simulink model "lineaEEC_prom"  (R2015a)
settings: Solver=ode45  StartTime=0.0  StopTime=0.1  RelTol=1e-3
values from neighbouring files (symbols this model uses):
  l0 = (0.002029 + 0.002392 + 0.002727 + 0.002296)/4    (= 0.002361)    [ParametrosTramo1.m]
  l1 = (0.001327 + 0.001263 + 0.001096 + 0.001311)/4    (= 0.00124925)    [ParametrosTramo1.m]
  Long = [0.26386 9.910026 3.09144 7.97976 2.97622 3.41433 1.495 4.41558 3.73037 10.41391 7.695292 4.39497 8.025209 3.99747 5.70753 10.31599 7.45101]'    [ParametrosTramo1.m]
  r0 = (0.4148+0.8307*3)/4    (= 0.726725)    [ParametrosTramo1.m]
  r1 = (0.4153+0.8315*3)/4    (= 0.72745)    [ParametrosTramo1.m]
libraries: powerlib x96
settings Model: CovSFcnEnable=off  Creator=ricardo  LastModifiedBy=USUARIO
settings DebuggingCC: SolverPrmCheckMsg=warning

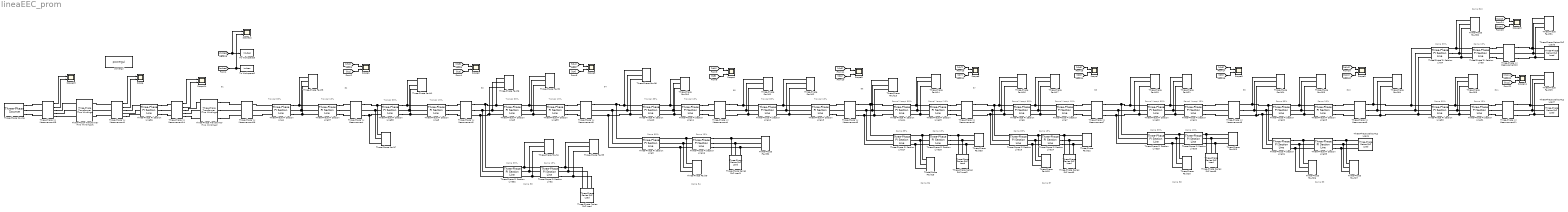
== system lineaEEC_prom ==
  note: B11
  note: B10
  note: B9
  note: B8
  note: B7
  note: B6
  note: B5
  note: B4
  note: Rama B3
  note: B3
  note: B2
  note: B1
  note: Rama 85%
  note: Troncal 85%
  note: Troncal 15%
  note: Rama 15%
  note: Troncal 85%
  note: Troncal 15%
  note: Troncal 85%
  note: Troncal 15%
  note: Troncal 85%
  note: Troncal 15%
  note: Troncal 85%
  note: Troncal 15%
  note: Rama 85%
  note: Rama 15%
  note: Rama 85%
  note: Rama 15%
  note: Ramal Yacopi 85%
  note: Ramal Yacopi 15%
  note: Ramal Yacopi 85%
  note: Ramal Yacopi 15%
  note: Ramal Yacopi 85%
  note: Ramal Yacopi 15%
  note: Rama 85%
  note: Rama 15%
  note: Rama 85%
  note: Rama 15%
  note: Rama 85%
  note: Rama 15%
  note: Rama 85%
  note: Rama 15%
  note: Rama 85%
  note: Rama 15%
  note: Rama B4
  note: Rama B6
  note: Rama B7
  note: Rama B8
  note: Rama B9
  note: Rama B10
  Scope{,1..12,14..15} (15 alike) : Scope  NumInputPorts=2
      Scope settings: YMin=-5~-5  YMax=5~5
      Scope1 settings: YMin=-5~-5  YMax=5~5
      Scope10 settings: YMin=-5~-5  YMax=5~5  SaveName=ScopeData10
      Scope11 settings: YMin=-5~-5  YMax=5~5  SaveName=ScopeData11
      Scope12 settings: TimeRange=0.03177083333333333  YMin=-4000~-5  YMax=4000~5  SaveName=ScopeData12
      Scope14 settings: YMin=-5~-5  YMax=5~5  SaveName=ScopeData14
      Scope15 settings: YMin=-175000~-1  YMax=100000~1.1  SaveName=ScopeData15
      Scope2 settings: YMin=-5~-5  YMax=5~5  SaveName=ScopeData2
      Scope3 settings: YMin=-5~-5  YMax=5~5  SaveName=ScopeData3
      Scope4 settings: YMin=-5~-5  YMax=5~5  SaveName=ScopeData4
      Scope5 settings: YMin=-5~-5  YMax=5~5  SaveName=ScopeData5
      Scope6 settings: YMin=-5~-5  YMax=5~5  SaveName=ScopeData6
      Scope7 settings: YMin=-5~-5  YMax=5~5  SaveName=ScopeData7
      Scope8 settings: YMin=-5~-5  YMax=5~5  SaveName=ScopeData8
      Scope9 settings: YMin=-5~-5  YMax=5~5  SaveName=ScopeData9
  Three-Phase PI Section Line1 : powerlib/Elements/Three-Phase PI Section Line  LConnTagsString=a|b|c  RConnTagsString=A|B|C  Frequency=60  Resistances=[ r1 r0]  Inductances="[ l1  l0]"  Capacitances=[12.74e-9 7.751e-9]  Length=Long(1)/2
  Three-Phase PI Section Line10 : powerlib/Elements/Three-Phase PI Section Line  LConnTagsString=a|b|c  RConnTagsString=A|B|C  Frequency=60  Resistances=[ r1 r0]  Inductances="[ l1  l0]"  Capacitances=[12.74e-9 7.751e-9]  Length=Long(4)/2
  Three-Phase PI Section Line11 : powerlib/Elements/Three-Phase PI Section Line  LConnTagsString=a|b|c  RConnTagsString=A|B|C  Frequency=60  Resistances=[ r1 r0]  Inductances="[ l1  l0]"  Capacitances=[12.74e-9 7.751e-9]  Length=Long(4)/2
  Three-Phase PI Section Line12 : powerlib/Elements/Three-Phase PI Section Line  LConnTagsString=a|b|c  RConnTagsString=A|B|C  Frequency=60  Resistances=[ r1 r0]  Inductances="[ l1  l0]"  Capacitances=[12.74e-9 7.751e-9]  Length=Long(5)/2
  Three-Phase PI Section Line13 : powerlib/Elements/Three-Phase PI Section Line  LConnTagsString=a|b|c  RConnTagsString=A|B|C  Frequency=60  Resistances=[ r1 r0]  Inductances="[ l1  l0]"  Capacitances=[12.74e-9 7.751e-9]  Length=Long(5)/2
  Three-Phase PI Section Line14 : powerlib/Elements/Three-Phase PI Section Line  LConnTagsString=a|b|c  RConnTagsString=A|B|C  Frequency=60  Resistances=[ r1 r0]  Inductances="[ l1  l0]"  Capacitances=[12.74e-9 7.751e-9]  Length=Long(6)/2
  Three-Phase PI Section Line15 : powerlib/Elements/Three-Phase PI Section Line  LConnTagsString=a|b|c  RConnTagsString=A|B|C  Frequency=60  Resistances=[ r1 r0]  Inductances="[ l1  l0]"  Capacitances=[12.74e-9 7.751e-9]  Length=Long(6)/2
  Three-Phase PI Section Line16 : powerlib/Elements/Three-Phase PI Section Line  LConnTagsString=a|b|c  RConnTagsString=A|B|C  Frequency=60  Resistances=[ r1 r0]  Inductances="[ l1  l0]"  Capacitances=[12.74e-9 7.751e-9]  Length=Long(12)/2
  Three-Phase PI Section Line17 : powerlib/Elements/Three-Phase PI Section Line  LConnTagsString=a|b|c  RConnTagsString=A|B|C  Frequency=60  Resistances=[ r1 r0]  Inductances="[ l1  l0]"  Capacitances=[12.74e-9 7.751e-9]  Length=Long(13)/2
  Three-Phase PI Section Line18 : powerlib/Elements/Three-Phase PI Section Line  LConnTagsString=a|b|c  RConnTagsString=A|B|C  Frequency=60  Resistances=[ r1 r0]  Inductances="[ l1  l0]"  Capacitances=[12.74e-9 7.751e-9]  Length=Long(13)/2
  Three-Phase PI Section Line19 : powerlib/Elements/Three-Phase PI Section Line  LConnTagsString=a|b|c  RConnTagsString=A|B|C  Frequency=60  Resistances=[ r1 r0]  Inductances="[ l1  l0]"  Capacitances=[12.74e-9 7.751e-9]  Length=Long(14)/2
  Three-Phase PI Section Line2 : powerlib/Elements/Three-Phase PI Section Line  LConnTagsString=a|b|c  RConnTagsString=A|B|C  Frequency=60  Resistances=[ r1 r0]  Inductances="[ l1  l0]"  Capacitances=[12.74e-9 7.751e-9]  Length=Long(11)/2
  Three-Phase PI Section Line20 : powerlib/Elements/Three-Phase PI Section Line  LConnTagsString=a|b|c  RConnTagsString=A|B|C  Frequency=60  Resistances=[ r1 r0]  Inductances="[ l1  l0]"  Capacitances=[12.74e-9 7.751e-9]  Length=Long(8)/2
  Three-Phase PI Section Line21 : powerlib/Elements/Three-Phase PI Section Line  LConnTagsString=a|b|c  RConnTagsString=A|B|C  Frequency=60  Resistances=[ r1 r0]  Inductances="[ l1  l0]"  Capacitances=[12.74e-9 7.751e-9]  Length=Long(8)/2
  Three-Phase PI Section Line22 : powerlib/Elements/Three-Phase PI Section Line  LConnTagsString=a|b|c  RConnTagsString=A|B|C  Frequency=60  Resistances=[ r1 r0]  Inductances="[ l1  l0]"  Capacitances=[12.74e-9 7.751e-9]  Length=Long(9)/2
  Three-Phase PI Section Line23 : powerlib/Elements/Three-Phase PI Section Line  LConnTagsString=a|b|c  RConnTagsString=A|B|C  Frequency=60  Resistances=[ r1 r0]  Inductances="[ l1  l0]"  Capacitances=[12.74e-9 7.751e-9]  Length=Long(9)/2
  Three-Phase PI Section Line24 : powerlib/Elements/Three-Phase PI Section Line  LConnTagsString=a|b|c  RConnTagsString=A|B|C  Frequency=60  Resistances=[ r1 r0]  Inductances="[ l1  l0]"  Capacitances=[12.74e-9 7.751e-9]  Length=Long(14)/2
  Three-Phase PI Section Line25 : powerlib/Elements/Three-Phase PI Section Line  LConnTagsString=a|b|c  RConnTagsString=A|B|C  Frequency=60  Resistances=[ r1 r0]  Inductances="[ l1  l0]"  Capacitances=[12.74e-9 7.751e-9]  Length=Long(15)/2
  Three-Phase PI Section Line3 : powerlib/Elements/Three-Phase PI Section Line  LConnTagsString=a|b|c  RConnTagsString=A|B|C  Frequency=60  Resistances=[ r1 r0]  Inductances="[ l1  l0]"  Capacitances=[12.74e-9 7.751e-9]  Length=Long(12)/2
  Three-Phase PI Section Line30 : powerlib/Elements/Three-Phase PI Section Line  LConnTagsString=a|b|c  RConnTagsString=A|B|C  Frequency=60  Resistances=[ r1 r0]  Inductances="[ l1  l0]"  Capacitances=[12.74e-9 7.751e-9]  Length=Long(10)/2
  Three-Phase PI Section Line31 : powerlib/Elements/Three-Phase PI Section Line  LConnTagsString=a|b|c  RConnTagsString=A|B|C  Frequency=60  Resistances=[ r1 r0]  Inductances="[ l1  l0]"  Capacitances=[12.74e-9 7.751e-9]  Length=Long(10)/2
  Three-Phase PI Section Line32 : powerlib/Elements/Three-Phase PI Section Line  LConnTagsString=a|b|c  RConnTagsString=A|B|C  Frequency=60  Resistances=[ r1 r0]  Inductances="[ l1  l0]"  Capacitances=[12.74e-9 7.751e-9]  Length=Long(11)/2
  Three-Phase PI Section Line33 : powerlib/Elements/Three-Phase PI Section Line  LConnTagsString=a|b|c  RConnTagsString=A|B|C  Frequency=60  Resistances=[ r1 r0]  Inductances="[ l1  l0]"  Capacitances=[12.74e-9 7.751e-9]  Length=Long(15)/2
  Three-Phase PI Section Line34 : powerlib/Elements/Three-Phase PI Section Line  LConnTagsString=a|b|c  RConnTagsString=A|B|C  Frequency=60  Resistances=[ r1 r0]  Inductances="[ l1  l0]"  Capacitances=[12.74e-9 7.751e-9]  Length=Long(16)/2
  Three-Phase PI Section Line35 : powerlib/Elements/Three-Phase PI Section Line  LConnTagsString=a|b|c  RConnTagsString=A|B|C  Frequency=60  Resistances=[ r1 r0]  Inductances="[ l1  l0]"  Capacitances=[12.74e-9 7.751e-9]  Length=Long(16)/2
  Three-Phase PI Section Line36 : powerlib/Elements/Three-Phase PI Section Line  LConnTagsString=a|b|c  RConnTagsString=A|B|C  Frequency=60  Resistances=[ 0.41586 0.82784]  Inductances="[ 1.3743e-3  4.2583e-3]"  Capacitances=[0.00825e-6 0.00588e-6]  Length=9
  Three-Phase PI Section Line37 : powerlib/Elements/Three-Phase PI Section Line  LConnTagsString=a|b|c  RConnTagsString=A|B|C  Frequency=60  Resistances=[ r1 r0]  Inductances="[ l1  l0]"  Capacitances=[12.74e-9 7.751e-9]  Length=Long(1)/2
  Three-Phase PI Section Line38 : powerlib/Elements/Three-Phase PI Section Line  LConnTagsString=a|b|c  RConnTagsString=A|B|C  Frequency=60  Resistances=[ r1 r0]  Inductances="[ l1  l0]"  Capacitances=[12.74e-9 7.751e-9]  Length=Long(2)/2
  Three-Phase PI Section Line39 : powerlib/Elements/Three-Phase PI Section Line  LConnTagsString=a|b|c  RConnTagsString=A|B|C  Frequency=60  Resistances=[ r1 r0]  Inductances="[ l1  l0]"  Capacitances=[12.74e-9 7.751e-9]  Length=Long(3)/2
  Three-Phase PI Section Line4 : powerlib/Elements/Three-Phase PI Section Line  LConnTagsString=a|b|c  RConnTagsString=A|B|C  Frequency=60  Resistances=[ r1 r0]  Inductances="[ l1  l0]"  Capacitances=[12.74e-9 7.751e-9]  Length=Long(17)/2
  Three-Phase PI Section Line5 : powerlib/Elements/Three-Phase PI Section Line  LConnTagsString=a|b|c  RConnTagsString=A|B|C  Frequency=60  Resistances=[ r1 r0]  Inductances="[ l1  l0]"  Capacitances=[12.74e-9 7.751e-9]  Length=Long(17)/2
  Three-Phase PI Section Line6 : powerlib/Elements/Three-Phase PI Section Line  LConnTagsString=a|b|c  RConnTagsString=A|B|C  Frequency=60  Resistances=[ r1 r0]  Inductances="[ l1  l0]"  Capacitances=[12.74e-9 7.751e-9]  Length=Long(7)/2
  Three-Phase PI Section Line7 : powerlib/Elements/Three-Phase PI Section Line  LConnTagsString=a|b|c  RConnTagsString=A|B|C  Frequency=60  Resistances=[ r1 r0]  Inductances="[ l1  l0]"  Capacitances=[12.74e-9 7.751e-9]  Length=Long(7)/2
  Three-Phase PI Section Line8 : powerlib/Elements/Three-Phase PI Section Line  LConnTagsString=a|b|c  RConnTagsString=A|B|C  Frequency=60  Resistances=[ r1 r0]  Inductances="[ l1  l0]"  Capacitances=[12.74e-9 7.751e-9]  Length=Long(2)/2
  Three-Phase PI Section Line9 : powerlib/Elements/Three-Phase PI Section Line  LConnTagsString=a|b|c  RConnTagsString=A|B|C  Frequency=60  Resistances=[ r1 r0]  Inductances="[ l1  l0]"  Capacitances=[12.74e-9 7.751e-9]  Length=Long(3)/2
  Three-Phase Series RLC Load : powerlib/Elements/Three-Phase Series RLC Load  LConnTagsString=A|B|C  Configuration=Y (grounded)  NominalVoltage=1000  NominalFrequency=60  ActivePower=7330  InductivePower=2140  CapacitivePower=0  Measurements=Branch voltages and currents  LoadType=constant PQ
  Three-Phase Series RLC Load1 : powerlib/Elements/Three-Phase Series RLC Load  LConnTagsString=A|B|C  Configuration=Y (grounded)  NominalVoltage=1000  NominalFrequency=60  ActivePower=16060  InductivePower=4690  CapacitivePower=0  Measurements=Branch voltages and currents  LoadType=constant PQ
  Three-Phase Series RLC Load2 : powerlib/Elements/Three-Phase Series RLC Load  LConnTagsString=A|B|C  Configuration=Y (grounded)  NominalVoltage=1000  NominalFrequency=60  ActivePower=5120  InductivePower=1490  CapacitivePower=0  Measurements=Branch voltages and currents  LoadType=constant PQ
  Three-Phase Series RLC Load3 : powerlib/Elements/Three-Phase Series RLC Load  LConnTagsString=A|B|C  Configuration=Y (grounded)  NominalVoltage=1000  NominalFrequency=60  ActivePower=10240  InductivePower=2990  CapacitivePower=0  Measurements=Branch voltages and currents  LoadType=constant PQ
  Three-Phase Series RLC Load4 : powerlib/Elements/Three-Phase Series RLC Load  LConnTagsString=A|B|C  Configuration=Y (grounded)  NominalVoltage=1000  NominalFrequency=60  ActivePower=9430  InductivePower=2750  CapacitivePower=0  Measurements=Branch voltages and currents  LoadType=constant PQ
  Three-Phase Series RLC Load5 : powerlib/Elements/Three-Phase Series RLC Load  LConnTagsString=A|B|C  Configuration=Y (grounded)  NominalVoltage=1000  NominalFrequency=60  ActivePower=28640  InductivePower=8350  CapacitivePower=0  Measurements=Branch voltages and currents  LoadType=constant PQ
  Three-Phase Series RLC Load6 : powerlib/Elements/Three-Phase Series RLC Load  LConnTagsString=A|B|C  Configuration=Y (grounded)  NominalVoltage=1000  NominalFrequency=60  ActivePower=10130  InductivePower=2950  CapacitivePower=0  Measurements=Branch voltages and currents  LoadType=constant PQ
  Three-Phase Series RLC Load7 : powerlib/Elements/Three-Phase Series RLC Load  LConnTagsString=A|B|C  Configuration=Y (grounded)  NominalVoltage=1000  NominalFrequency=60  ActivePower=6980  InductivePower=2040  CapacitivePower=0  Measurements=Branch voltages and currents  LoadType=constant PQ
  Three-Phase Transformer (Two Windings) : powerlib/Elements/Three-Phase Transformer (Two Windings)  Winding1Connection=Yg  Winding2Connection=Yg  CoreType=Three single-phase transformers  SetSaturation=off  Hysteresis=off  DataFile='hysteresis'  SetInitialFlux=off  Measurements=None  UNITS=pu  NominalPower=[ 5e6 , 60 ]  Winding1=[ 34500 , 0 , 0.0273 ]  Winding2=[ 13500 , 0 , 0.0273 ]  Rm=500  Lm=500  L0=0.5  Saturation=[ 0,0 ; 0.0024,1.2 ; 1.0,1.52 ]  InitialFluxes=[ 0.8 , -0.8 , 0.7 ]  MoreParameters=off  BreakLoop=off  DataType=off  TransfoNumber=1
  Three-Phase Transformer (Two Windings)1 : powerlib/Elements/Three-Phase Transformer (Two Windings)  Winding1Connection=Yg  Winding2Connection=Yg  CoreType=Three single-phase transformers  SetSaturation=off  Hysteresis=off  DataFile='hysteresis'  SetInitialFlux=off  Measurements=None  UNITS=pu  NominalPower=[ 40e6 , 60 ]  Winding1=[ 115000 , 0 , 0.06 ]  Winding2=[ 34500 , 0 , 0.06 ]  Rm=500  Lm=500  L0=0.5  Saturation=[ 0,0 ; 0.0024,1.2 ; 1.0,1.52 ]  InitialFluxes=[ 0.8 , -0.8 , 0.7 ]  MoreParameters=off  BreakLoop=off  DataType=off  TransfoNumber=1
  Three-Phase V-I Measurement : powerlib/Measurements/Three-Phase V-I Measurement  VoltageMeasurement=phase-to-phase  SetLabelV=on  LabelV=Vb2  Vpu=off  VpuLL=off  CurrentMeasurement=yes  SetLabelI=on  LabelI=Ib2  Ipu=off  Pbase=100e6  Vbase=500e3  OutputType=Complex  PhasorSimulation=off  PSBequivalent=0
  Three-Phase V-I Measurement1 : powerlib/Measurements/Three-Phase V-I Measurement  VoltageMeasurement=phase-to-phase  SetLabelV=off  LabelV=Vabc  Vpu=off  VpuLL=off  CurrentMeasurement=yes  SetLabelI=off  LabelI=Iabc  Ipu=off  Pbase=100e6  Vbase=500e3  OutputType=Complex  PhasorSimulation=off  PSBequivalent=0
  Three-Phase V-I Measurement10 : powerlib/Measurements/Three-Phase V-I Measurement  VoltageMeasurement=phase-to-phase  SetLabelV=on  LabelV=Vb10r  Vpu=off  VpuLL=off  CurrentMeasurement=yes  SetLabelI=on  LabelI=Ib10r  Ipu=off  Pbase=100e6  Vbase=500e3  OutputType=Complex  PhasorSimulation=off  PSBequivalent=0
  Three-Phase V-I Measurement11 : powerlib/Measurements/Three-Phase V-I Measurement  VoltageMeasurement=phase-to-phase  SetLabelV=on  LabelV=Vb11  Vpu=off  VpuLL=off  CurrentMeasurement=yes  SetLabelI=on  LabelI=Ib11  Ipu=off  Pbase=100e6  Vbase=500e3  OutputType=Complex  PhasorSimulation=off  PSBequivalent=0
  Three-Phase V-I Measurement14 : powerlib/Measurements/Three-Phase V-I Measurement  VoltageMeasurement=phase-to-phase  SetLabelV=off  LabelV=Vabc  Vpu=off  VpuLL=off  CurrentMeasurement=yes  SetLabelI=off  LabelI=Iabc  Ipu=off  Pbase=100e6  Vbase=500e3  OutputType=Complex  PhasorSimulation=off  PSBequivalent=0
  Three-Phase V-I Measurement15 : powerlib/Measurements/Three-Phase V-I Measurement  VoltageMeasurement=phase-to-phase  SetLabelV=off  LabelV=Vabc  Vpu=off  VpuLL=off  CurrentMeasurement=yes  SetLabelI=off  LabelI=Iabc  Ipu=off  Pbase=100e6  Vbase=500e3  OutputType=Complex  PhasorSimulation=off  PSBequivalent=0
  Three-Phase V-I Measurement16 : powerlib/Measurements/Three-Phase V-I Measurement  VoltageMeasurement=phase-to-phase  SetLabelV=on  LabelV=Vsubes  Vpu=off  VpuLL=off  CurrentMeasurement=yes  SetLabelI=on  LabelI=Isubes  Ipu=off  Pbase=100e6  Vbase=500e3  OutputType=Complex  PhasorSimulation=off  PSBequivalent=0
  Three-Phase V-I Measurement2 : powerlib/Measurements/Three-Phase V-I Measurement  VoltageMeasurement=phase-to-phase  SetLabelV=on  LabelV=Vb3  Vpu=off  VpuLL=off  CurrentMeasurement=yes  SetLabelI=on  LabelI=Ib3  Ipu=off  Pbase=100e6  Vbase=500e3  OutputType=Complex  PhasorSimulation=off  PSBequivalent=0
  Three-Phase V-I Measurement3 : powerlib/Measurements/Three-Phase V-I Measurement  VoltageMeasurement=phase-to-phase  SetLabelV=on  LabelV=Vb4  Vpu=off  VpuLL=off  CurrentMeasurement=yes  SetLabelI=on  LabelI=Ib4  Ipu=off  Pbase=100e6  Vbase=500e3  OutputType=Complex  PhasorSimulation=off  PSBequivalent=0
  Three-Phase V-I Measurement4 : powerlib/Measurements/Three-Phase V-I Measurement  VoltageMeasurement=phase-to-phase  SetLabelV=on  LabelV=Vb5  Vpu=off  VpuLL=off  CurrentMeasurement=yes  SetLabelI=on  LabelI=Ib5  Ipu=off  Pbase=100e6  Vbase=500e3  OutputType=Complex  PhasorSimulation=off  PSBequivalent=0
  Three-Phase V-I Measurement5 : powerlib/Measurements/Three-Phase V-I Measurement  VoltageMeasurement=phase-to-phase  SetLabelV=on  LabelV=Vb6  Vpu=off  VpuLL=off  CurrentMeasurement=yes  SetLabelI=on  LabelI=Ib6  Ipu=off  Pbase=100e6  Vbase=500e3  OutputType=Complex  PhasorSimulation=off  PSBequivalent=0
  Three-Phase V-I Measurement6 : powerlib/Measurements/Three-Phase V-I Measurement  VoltageMeasurement=phase-to-phase  SetLabelV=on  LabelV=Vb7  Vpu=off  VpuLL=off  CurrentMeasurement=yes  SetLabelI=on  LabelI=Ib7  Ipu=off  Pbase=100e6  Vbase=500e3  OutputType=Complex  PhasorSimulation=off  PSBequivalent=0
  Three-Phase V-I Measurement7 : powerlib/Measurements/Three-Phase V-I Measurement  VoltageMeasurement=phase-to-phase  SetLabelV=on  LabelV=Vb8  Vpu=off  VpuLL=off  CurrentMeasurement=yes  SetLabelI=on  LabelI=Ib8  Ipu=off  Pbase=100e6  Vbase=500e3  OutputType=Complex  PhasorSimulation=off  PSBequivalent=0
  Three-Phase V-I Measurement8 : powerlib/Measurements/Three-Phase V-I Measurement  VoltageMeasurement=phase-to-phase  SetLabelV=on  LabelV=Vb9  Vpu=off  VpuLL=off  CurrentMeasurement=yes  SetLabelI=on  LabelI=Ib9  Ipu=off  Pbase=100e6  Vbase=500e3  OutputType=Complex  PhasorSimulation=off  PSBequivalent=0
  Three-Phase V-I Measurement9 : powerlib/Measurements/Three-Phase V-I Measurement  VoltageMeasurement=phase-to-phase  SetLabelV=on  LabelV=Vb10  Vpu=off  VpuLL=off  CurrentMeasurement=yes  SetLabelI=on  LabelI=Ib10  Ipu=off  Pbase=100e6  Vbase=500e3  OutputType=Complex  PhasorSimulation=off  PSBequivalent=0
  Three-Phase Fault{1..34} (34 alike) : powerlib/Elements/Three-Phase Fault  InitialStates=0  FaultA=off  FaultB=off  FaultC=off  GroundFault=off  SwitchTimes="[3/60  6/60]"  External=off  SwitchStatus=NaN  FaultResistance=0.001  GroundResistance=0.01  SnubberResistance=1e6  SnubberCapacitance=inf  Measurements=None
  Three-Phase Source : powerlib/Electrical Sources/Three-Phase Source  Voltage=115000  PhaseAngle=0  Frequency=60  InternalConnection=Yg  SpecifyImpedance=on  Resistance=0.8929  Inductance=16.58e-3  ShortCircuitLevel=100e6  BaseVoltage=115000  XRratio=7  BusType=swing  Pref=0  Qref=0  Qmin=-inf  Qmax=inf
  To Workspace2 : ToWorkspace  VariableName=Isubes  SampleTime=-1
  To Workspace3 : ToWorkspace  VariableName=Vsubes  SampleTime=-1
  powergui : powerlib/powergui  Priority=1  SimulationMode=Discrete  SolverType=Tustin  SampleTime=5.208333e-4  frequency=60  SPID=off  DisableSnubberDevices=off  DisableRonSwitches=off  DisableVfSwitches=off  SwTol=0  DisplayEquations=off  Interpol=off  methode=off  Ts=0  FunctionMessages=off  echomessages=off  HookPort=off  EnableUseOfTLC=off  x0status=blocks  frequencyindice=60  Pbase=100e6  ErrMax=1e-4  Iterations=100  UnitsV=kV  UnitsW=MW  buscounter=0  RestoreLinks=warning  ResistiveCurrentMeasurement=off  Frange=[0:2:500]  Ylog=off  Xlog=on  ShowGrid=off  save=off  variable=ZData  structure=0  ZoomFFT=off  StartTime=0.0  cycles=1  DisplayStyle=1  fundamental=60  FreqAxis=off  MaxFrequency=1000  frequencyindicesteady=1  RmsSteady=1  display=off
  wires:
  Three-Phase V-I Measurement14/2 -> Scope14/2
  Three-Phase V-I Measurement14/1 -> Scope14/1
  Three-Phase V-I Measurement1/1 -> Scope/1
  Three-Phase V-I Measurement1/2 -> Scope/2
  Three-Phase V-I Measurement15/1 -> Scope15/1
  Three-Phase V-I Measurement15/2 -> Scope15/2
  [Vsubes] -> Scope12/1, To Workspace3/1
  [Isubes] -> Scope12/2, To Workspace2/1
  [Vb2] -> Scope1/1
  [Ib2] -> Scope1/2
  [Vb3] -> Scope2/1
  [Ib3] -> Scope2/2
  [Vb4] -> Scope3/1
  [Ib4] -> Scope3/2
  [Vb5] -> Scope4/1
  [Ib5] -> Scope4/2
  [Vb6] -> Scope5/1
  [Ib6] -> Scope5/2
  [Vb7] -> Scope6/1
  [Ib7] -> Scope6/2
  [Vb8] -> Scope7/1
  [Ib8] -> Scope7/2
  [Vb9] -> Scope8/1
  [Ib9] -> Scope8/2
  [Vb10] -> Scope9/1
  [Ib10] -> Scope9/2
  [Vb11] -> Scope11/1
  [Ib11] -> Scope11/2
  [Vb10r] -> Scope10/1
  [Ib10r] -> Scope10/2
  connections:
  Three-Phase PI Section Line39/LConn2 -- Three-Phase PI Section Line9/RConn2 -- Three-Phase Fault2/LConn2
  Three-Phase PI Section Line39/LConn3 -- Three-Phase PI Section Line9/RConn3 -- Three-Phase Fault2/LConn3
  Three-Phase PI Section Line39/LConn1 -- Three-Phase PI Section Line9/RConn1 -- Three-Phase Fault2/LConn1
  Three-Phase PI Section Line11/LConn2 -- Three-Phase PI Section Line10/RConn2 -- Three-Phase Fault10/LConn2
  Three-Phase PI Section Line11/LConn3 -- Three-Phase PI Section Line10/RConn3 -- Three-Phase Fault10/LConn3
  Three-Phase PI Section Line11/LConn1 -- Three-Phase Fault10/LConn1 -- Three-Phase PI Section Line10/RConn1
  Three-Phase PI Section Line13/LConn2 -- Three-Phase Fault12/LConn2 -- Three-Phase PI Section Line12/RConn2
  Three-Phase PI Section Line13/LConn3 -- Three-Phase Fault12/LConn3 -- Three-Phase PI Section Line12/RConn3
  Three-Phase PI Section Line13/LConn1 -- Three-Phase Fault12/LConn1 -- Three-Phase PI Section Line12/RConn1
  Three-Phase PI Section Line2/LConn1 -- Three-Phase Fault4/LConn1 -- Three-Phase PI Section Line32/RConn1
  Three-Phase PI Section Line2/LConn2 -- Three-Phase Fault4/LConn2 -- Three-Phase PI Section Line32/RConn2
  Three-Phase PI Section Line2/LConn3 -- Three-Phase Fault4/LConn3 -- Three-Phase PI Section Line32/RConn3
  Three-Phase PI Section Line16/LConn2 -- Three-Phase Fault9/LConn2 -- Three-Phase PI Section Line3/RConn2
  Three-Phase PI Section Line16/RConn1 -- Three-Phase Fault32/LConn1 -- Three-Phase Series RLC Load1/LConn1
  Three-Phase PI Section Line16/RConn2 -- Three-Phase Fault32/LConn2 -- Three-Phase Series RLC Load1/LConn2
  Three-Phase PI Section Line16/RConn3 -- Three-Phase Fault32/LConn3 -- Three-Phase Series RLC Load1/LConn3
  Three-Phase PI Section Line16/LConn3 -- Three-Phase Fault9/LConn3 -- Three-Phase PI Section Line3/RConn3
  Three-Phase PI Section Line16/LConn1 -- Three-Phase Fault9/LConn1 -- Three-Phase PI Section Line3/RConn1
  Three-Phase PI Section Line18/RConn1 -- Three-Phase Fault33/LConn1 -- Three-Phase Series RLC Load2/LConn1
  Three-Phase PI Section Line18/LConn3 -- Three-Phase Fault15/LConn3 -- Three-Phase PI Section Line17/RConn3
  Three-Phase PI Section Line18/LConn1 -- Three-Phase Fault15/LConn1 -- Three-Phase PI Section Line17/RConn1
  Three-Phase PI Section Line18/LConn2 -- Three-Phase Fault15/LConn2 -- Three-Phase PI Section Line17/RConn2
  Three-Phase PI Section Line18/RConn2 -- Three-Phase Fault33/LConn2 -- Three-Phase Series RLC Load2/LConn2
  Three-Phase PI Section Line18/RConn3 -- Three-Phase Fault33/LConn3 -- Three-Phase Series RLC Load2/LConn3
  Three-Phase PI Section Line24/LConn2 -- Three-Phase Fault18/LConn2 -- Three-Phase PI Section Line19/RConn2
  Three-Phase PI Section Line24/LConn3 -- Three-Phase Fault18/LConn3 -- Three-Phase PI Section Line19/RConn3
  Three-Phase PI Section Line24/RConn2 -- Three-Phase Fault22/LConn2 -- Three-Phase Series RLC Load3/LConn2
  Three-Phase PI Section Line24/LConn1 -- Three-Phase Fault18/LConn1 -- Three-Phase PI Section Line19/RConn1
  Three-Phase PI Section Line24/RConn3 -- Three-Phase Fault22/LConn3 -- Three-Phase Series RLC Load3/LConn3
  Three-Phase PI Section Line24/RConn1 -- Three-Phase Fault22/LConn1 -- Three-Phase Series RLC Load3/LConn1
  Three-Phase PI Section Line15/LConn1 -- Three-Phase Fault14/LConn1 -- Three-Phase PI Section Line14/RConn1
  Three-Phase PI Section Line15/LConn2 -- Three-Phase Fault14/LConn2 -- Three-Phase PI Section Line14/RConn2
  Three-Phase PI Section Line15/LConn3 -- Three-Phase Fault14/LConn3 -- Three-Phase PI Section Line14/RConn3
  Three-Phase PI Section Line7/LConn1 -- Three-Phase Fault17/LConn1 -- Three-Phase PI Section Line6/RConn1
  Three-Phase PI Section Line7/LConn2 -- Three-Phase Fault17/LConn2 -- Three-Phase PI Section Line6/RConn2
  Three-Phase PI Section Line7/LConn3 -- Three-Phase Fault17/LConn3 -- Three-Phase PI Section Line6/RConn3
  Three-Phase PI Section Line21/LConn1 -- Three-Phase Fault21/LConn1 -- Three-Phase PI Section Line20/RConn1
  Three-Phase PI Section Line21/LConn2 -- Three-Phase Fault21/LConn2 -- Three-Phase PI Section Line20/RConn2
  Three-Phase PI Section Line21/LConn3 -- Three-Phase Fault21/LConn3 -- Three-Phase PI Section Line20/RConn3
  Three-Phase PI Section Line33/RConn1 -- Three-Phase Fault23/LConn1 -- Three-Phase Series RLC Load5/LConn1
  Three-Phase PI Section Line33/RConn2 -- Three-Phase Fault23/LConn2 -- Three-Phase Series RLC Load5/LConn2
  Three-Phase PI Section Line33/RConn3 -- Three-Phase Fault23/LConn3 -- Three-Phase Series RLC Load5/LConn3
  Three-Phase PI Section Line23/LConn1 -- Three-Phase Fault25/LConn1 -- Three-Phase PI Section Line22/RConn1
  Three-Phase PI Section Line23/LConn2 -- Three-Phase Fault25/LConn2 -- Three-Phase PI Section Line22/RConn2
  Three-Phase PI Section Line23/LConn3 -- Three-Phase Fault25/LConn3 -- Three-Phase PI Section Line22/RConn3
  Three-Phase PI Section Line31/LConn2 -- Three-Phase Fault28/LConn2 -- Three-Phase PI Section Line30/RConn2
  Three-Phase PI Section Line31/LConn3 -- Three-Phase Fault28/LConn3 -- Three-Phase PI Section Line30/RConn3
  Three-Phase PI Section Line31/LConn1 -- Three-Phase Fault28/LConn1 -- Three-Phase PI Section Line30/RConn1
  Three-Phase PI Section Line33/LConn3 -- Three-Phase Fault20/LConn3 -- Three-Phase PI Section Line25/RConn3
  Three-Phase PI Section Line33/LConn2 -- Three-Phase Fault20/LConn2 -- Three-Phase PI Section Line25/RConn2
  Three-Phase PI Section Line33/LConn1 -- Three-Phase Fault20/LConn1 -- Three-Phase PI Section Line25/RConn1
  Three-Phase PI Section Line4/RConn2 -- Three-Phase Fault30/LConn2 -- Three-Phase PI Section Line5/LConn2
  Three-Phase PI Section Line5/LConn3 -- Three-Phase Fault30/LConn3 -- Three-Phase PI Section Line4/RConn3
  Three-Phase PI Section Line5/LConn1 -- Three-Phase Fault30/LConn1 -- Three-Phase PI Section Line4/RConn1
  Three-Phase PI Section Line37/RConn1 -- Three-Phase V-I Measurement/LConn1
  Three-Phase PI Section Line37/RConn2 -- Three-Phase V-I Measurement/LConn2
  Three-Phase PI Section Line37/RConn3 -- Three-Phase V-I Measurement/LConn3
  Three-Phase PI Section Line8/RConn1 -- Three-Phase V-I Measurement2/LConn1
  Three-Phase PI Section Line8/RConn2 -- Three-Phase V-I Measurement2/LConn2
  Three-Phase PI Section Line8/RConn3 -- Three-Phase V-I Measurement2/LConn3
  Three-Phase PI Section Line39/RConn1 -- Three-Phase V-I Measurement3/LConn1
  Three-Phase PI Section Line39/RConn2 -- Three-Phase V-I Measurement3/LConn2
  Three-Phase PI Section Line39/RConn3 -- Three-Phase V-I Measurement3/LConn3
  Three-Phase PI Section Line11/RConn1 -- Three-Phase V-I Measurement4/LConn1
  Three-Phase PI Section Line11/RConn2 -- Three-Phase V-I Measurement4/LConn2
  Three-Phase PI Section Line11/RConn3 -- Three-Phase V-I Measurement4/LConn3
  Three-Phase PI Section Line15/RConn1 -- Three-Phase V-I Measurement6/LConn1
  Three-Phase PI Section Line15/RConn2 -- Three-Phase V-I Measurement6/LConn2
  Three-Phase PI Section Line15/RConn3 -- Three-Phase V-I Measurement6/LConn3
  Three-Phase PI Section Line31/RConn1 -- Three-Phase V-I Measurement11/LConn1
  Three-Phase PI Section Line31/RConn2 -- Three-Phase V-I Measurement11/LConn2
  Three-Phase PI Section Line31/RConn3 -- Three-Phase V-I Measurement11/LConn3
  Three-Phase V-I Measurement1/LConn2 -- Three-Phase Transformer (Two Windings)1/RConn2
  Three-Phase V-I Measurement1/LConn1 -- Three-Phase Transformer (Two Windings)1/RConn1
  Three-Phase V-I Measurement1/LConn3 -- Three-Phase Transformer (Two Windings)1/RConn3
  Three-Phase PI Section Line36/RConn3 -- Three-Phase V-I Measurement14/LConn3
  Three-Phase PI Section Line36/RConn2 -- Three-Phase V-I Measurement14/LConn2
  Three-Phase PI Section Line36/RConn1 -- Three-Phase V-I Measurement14/LConn1
  Three-Phase V-I Measurement1/RConn1 -- Three-Phase PI Section Line36/LConn1
  Three-Phase PI Section Line36/LConn2 -- Three-Phase V-I Measurement1/RConn2
  Three-Phase V-I Measurement1/RConn3 -- Three-Phase PI Section Line36/LConn3
  Three-Phase V-I Measurement14/RConn3 -- Three-Phase Transformer (Two Windings)/LConn3
  Three-Phase V-I Measurement14/RConn2 -- Three-Phase Transformer (Two Windings)/LConn2
  Three-Phase V-I Measurement14/RConn1 -- Three-Phase Transformer (Two Windings)/LConn1
  Three-Phase Source/RConn2 -- Three-Phase V-I Measurement15/LConn2
  Three-Phase Source/RConn1 -- Three-Phase V-I Measurement15/LConn1
  Three-Phase Source/RConn3 -- Three-Phase V-I Measurement15/LConn3
  Three-Phase V-I Measurement15/RConn3 -- Three-Phase Transformer (Two Windings)1/LConn3
  Three-Phase V-I Measurement15/RConn2 -- Three-Phase Transformer (Two Windings)1/LConn2
  Three-Phase V-I Measurement15/RConn1 -- Three-Phase Transformer (Two Windings)1/LConn1
  Three-Phase Transformer (Two Windings)/RConn2 -- Three-Phase V-I Measurement16/LConn2
  Three-Phase Transformer (Two Windings)/RConn1 -- Three-Phase V-I Measurement16/LConn1
  Three-Phase Transformer (Two Windings)/RConn3 -- Three-Phase V-I Measurement16/LConn3
  Three-Phase PI Section Line1/LConn1 -- Three-Phase V-I Measurement16/RConn1
  Three-Phase PI Section Line1/LConn2 -- Three-Phase V-I Measurement16/RConn2
  Three-Phase PI Section Line1/LConn3 -- Three-Phase V-I Measurement16/RConn3
  Three-Phase PI Section Line1/RConn1 -- Three-Phase Fault3/LConn1 -- Three-Phase PI Section Line37/LConn1
  Three-Phase PI Section Line37/LConn2 -- Three-Phase Fault3/LConn2 -- Three-Phase PI Section Line1/RConn2
  Three-Phase PI Section Line1/RConn3 -- Three-Phase Fault3/LConn3 -- Three-Phase PI Section Line37/LConn3
  Three-Phase PI Section Line38/RConn1 -- Three-Phase Fault1/LConn1 -- Three-Phase PI Section Line8/LConn1
  Three-Phase PI Section Line8/LConn2 -- Three-Phase Fault1/LConn2 -- Three-Phase PI Section Line38/RConn2
  Three-Phase PI Section Line38/RConn3 -- Three-Phase Fault1/LConn3 -- Three-Phase PI Section Line8/LConn3
  Three-Phase PI Section Line34/RConn1 -- Three-Phase Fault26/LConn1 -- Three-Phase PI Section Line35/LConn1
  Three-Phase PI Section Line35/LConn2 -- Three-Phase Fault26/LConn2 -- Three-Phase PI Section Line34/RConn2
  Three-Phase PI Section Line34/RConn3 -- Three-Phase Fault26/LConn3 -- Three-Phase PI Section Line35/LConn3
  Three-Phase V-I Measurement/RConn1 -- Three-Phase Fault7/LConn1 -- Three-Phase PI Section Line38/LConn1
  Three-Phase PI Section Line38/LConn2 -- Three-Phase Fault7/LConn2 -- Three-Phase V-I Measurement/RConn2
  Three-Phase V-I Measurement/RConn3 -- Three-Phase Fault7/LConn3 -- Three-Phase PI Section Line38/LConn3
  Three-Phase V-I Measurement2/RConn1 -- Three-Phase PI Section Line32/LConn1 -- Three-Phase Fault6/LConn1 -- Three-Phase PI Section Line9/LConn1
  Three-Phase V-I Measurement2/RConn2 -- Three-Phase PI Section Line32/LConn2 -- Three-Phase Fault6/LConn2 -- Three-Phase PI Section Line9/LConn2
  Three-Phase PI Section Line9/LConn3 -- Three-Phase Fault6/LConn3 -- Three-Phase PI Section Line32/LConn3 -- Three-Phase V-I Measurement2/RConn3
  Three-Phase V-I Measurement3/RConn1 -- Three-Phase PI Section Line3/LConn1 -- Three-Phase Fault8/LConn1 -- Three-Phase PI Section Line10/LConn1
  Three-Phase PI Section Line10/LConn2 -- Three-Phase Fault8/LConn2 -- Three-Phase PI Section Line3/LConn2 -- Three-Phase V-I Measurement3/RConn2
  Three-Phase PI Section Line10/LConn3 -- Three-Phase Fault8/LConn3 -- Three-Phase PI Section Line3/LConn3 -- Three-Phase V-I Measurement3/RConn3
  Three-Phase PI Section Line2/RConn1 -- Three-Phase Fault5/LConn1 -- Three-Phase Series RLC Load/LConn1
  Three-Phase Series RLC Load/LConn2 -- Three-Phase Fault5/LConn2 -- Three-Phase PI Section Line2/RConn2
  Three-Phase PI Section Line2/RConn3 -- Three-Phase Fault5/LConn3 -- Three-Phase Series RLC Load/LConn3
  Three-Phase V-I Measurement4/RConn1 -- Three-Phase Fault11/LConn1 -- Three-Phase PI Section Line12/LConn1
  Three-Phase V-I Measurement4/RConn2 -- Three-Phase Fault11/LConn2 -- Three-Phase PI Section Line12/LConn2
  Three-Phase PI Section Line12/LConn3 -- Three-Phase Fault11/LConn3 -- Three-Phase V-I Measurement4/RConn3
  Three-Phase V-I Measurement5/LConn1 -- Three-Phase PI Section Line13/RConn1
  Three-Phase V-I Measurement5/LConn2 -- Three-Phase PI Section Line13/RConn2
  Three-Phase PI Section Line13/RConn3 -- Three-Phase V-I Measurement5/LConn3
  Three-Phase V-I Measurement5/RConn1 -- Three-Phase PI Section Line17/LConn1 -- Three-Phase Fault13/LConn1 -- Three-Phase PI Section Line14/LConn1
  Three-Phase PI Section Line14/LConn2 -- Three-Phase Fault13/LConn2 -- Three-Phase PI Section Line17/LConn2 -- Three-Phase V-I Measurement5/RConn2
  Three-Phase V-I Measurement5/RConn3 -- Three-Phase PI Section Line17/LConn3 -- Three-Phase Fault13/LConn3 -- Three-Phase PI Section Line14/LConn3
  Three-Phase V-I Measurement6/RConn1 -- Three-Phase PI Section Line19/LConn1 -- Three-Phase Fault16/LConn1 -- Three-Phase PI Section Line6/LConn1
  Three-Phase PI Section Line6/LConn2 -- Three-Phase Fault16/LConn2 -- Three-Phase PI Section Line19/LConn2 -- Three-Phase V-I Measurement6/RConn2
  Three-Phase PI Section Line6/LConn3 -- Three-Phase Fault16/LConn3 -- Three-Phase PI Section Line19/LConn3 -- Three-Phase V-I Measurement6/RConn3
  Three-Phase PI Section Line7/RConn1 -- Three-Phase V-I Measurement7/LConn1
  Three-Phase V-I Measurement7/LConn2 -- Three-Phase PI Section Line7/RConn2
  Three-Phase PI Section Line7/RConn3 -- Three-Phase V-I Measurement7/LConn3
  Three-Phase V-I Measurement7/RConn1 -- Three-Phase PI Section Line25/LConn1 -- Three-Phase Fault19/LConn1 -- Three-Phase PI Section Line20/LConn1
  Three-Phase PI Section Line20/LConn2 -- Three-Phase Fault19/LConn2 -- Three-Phase PI Section Line25/LConn2 -- Three-Phase V-I Measurement7/RConn2
  Three-Phase V-I Measurement7/RConn3 -- Three-Phase PI Section Line25/LConn3 -- Three-Phase Fault19/LConn3 -- Three-Phase PI Section Line20/LConn3
  Three-Phase PI Section Line21/RConn1 -- Three-Phase V-I Measurement8/LConn1
  Three-Phase V-I Measurement8/LConn2 -- Three-Phase PI Section Line21/RConn2
  Three-Phase PI Section Line21/RConn3 -- Three-Phase V-I Measurement8/LConn3
  Three-Phase PI Section Line35/RConn1 -- Three-Phase Fault27/LConn1 -- Three-Phase Series RLC Load4/LConn1
  Three-Phase Series RLC Load4/LConn2 -- Three-Phase Fault27/LConn2 -- Three-Phase PI Section Line35/RConn2
  Three-Phase PI Section Line35/RConn3 -- Three-Phase Fault27/LConn3 -- Three-Phase Series RLC Load4/LConn3
  Three-Phase PI Section Line22/LConn1 -- Three-Phase PI Section Line34/LConn1 -- Three-Phase Fault24/LConn1 -- Three-Phase V-I Measurement8/RConn1
  Three-Phase V-I Measurement8/RConn2 -- Three-Phase Fault24/LConn2 -- Three-Phase PI Section Line34/LConn2 -- Three-Phase PI Section Line22/LConn2
  Three-Phase PI Section Line22/LConn3 -- Three-Phase PI Section Line34/LConn3 -- Three-Phase Fault24/LConn3 -- Three-Phase V-I Measurement8/RConn3
  Three-Phase PI Section Line23/RConn1 -- Three-Phase V-I Measurement9/LConn1
  Three-Phase V-I Measurement9/LConn2 -- Three-Phase PI Section Line23/RConn2
  Three-Phase PI Section Line23/RConn3 -- Three-Phase V-I Measurement9/LConn3
  Three-Phase V-I Measurement9/RConn1 -- Three-Phase Fault34/LConn1 -- Three-Phase PI Section Line4/LConn1 -- Three-Phase PI Section Line30/LConn1
  Three-Phase V-I Measurement9/RConn2 -- Three-Phase Fault34/LConn2 -- Three-Phase PI Section Line4/LConn2 -- Three-Phase PI Section Line30/LConn2
  Three-Phase V-I Measurement9/RConn3 -- Three-Phase Fault34/LConn3 -- Three-Phase PI Section Line4/LConn3 -- Three-Phase PI Section Line30/LConn3
  Three-Phase V-I Measurement11/RConn1 -- Three-Phase Fault29/LConn1 -- Three-Phase Series RLC Load7/LConn1
  Three-Phase Series RLC Load7/LConn2 -- Three-Phase Fault29/LConn2 -- Three-Phase V-I Measurement11/RConn2
  Three-Phase V-I Measurement11/RConn3 -- Three-Phase Fault29/LConn3 -- Three-Phase Series RLC Load7/LConn3
  Three-Phase PI Section Line5/RConn1 -- Three-Phase V-I Measurement10/LConn1
  Three-Phase V-I Measurement10/LConn2 -- Three-Phase PI Section Line5/RConn2
  Three-Phase PI Section Line5/RConn3 -- Three-Phase V-I Measurement10/LConn3
  Three-Phase V-I Measurement10/RConn1 -- Three-Phase Fault31/LConn1 -- Three-Phase Series RLC Load6/LConn1
  Three-Phase Series RLC Load6/LConn2 -- Three-Phase Fault31/LConn2 -- Three-Phase V-I Measurement10/RConn2
  Three-Phase V-I Measurement10/RConn3 -- Three-Phase Fault31/LConn3 -- Three-Phase Series RLC Load6/LConn3
